simulink model "ResidualsGen"  (Simulink 9.3)
settings: Solver=ode23tb  StartTime=0.0  StopTime=1219  EnableMultiTasking=on
values from neighbouring files (symbols this model uses):
  omega_min = TC_ENGINE.turbo.omega_min    [RunEngine.m]
settings Model: Creator=nkymark  LastModifiedBy=markng
settings SolverCC: MaxConsecutiveMinStep=100  ZeroCrossControl=EnableAll  SolverResetMethod=Robust
settings DataIOCC: LimitDataPoints=on
settings DebuggingCC: AllowSymbolicDim=off  PregeneratedLibrarySubsystemCodeDiagnostic=none
settings SFSimCC: SimParseCustomCode=off
settings GRTTargetCC: GeneratePreprocessorConditionals=Disable all

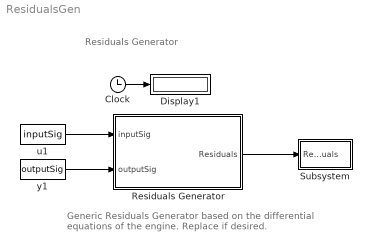
== system ResidualsGen ==
  note: Residuals Generator
  note: Generic Residuals Generator based on the differential
      | equations of the engine. Replace if desired.
  Clock : Clock
  Display1 : Display
  Residuals Generator : Subsystem
  Subsystem : Subsystem
  u1 : FromWorkspace  VariableName=inputSig  SampleTime=0
  y1 : FromWorkspace  VariableName=outputSig  SampleTime=0
  wires:
  Clock/1 -> Display1/1
  Residuals Generator/1(Residuals) -> Subsystem/1(Residuals)
  y1/1 -> Residuals Generator/2(outputSig)
  u1/1 -> Residuals Generator/1(inputSig)

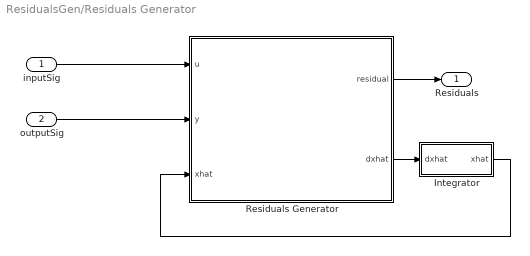
== system ResidualsGen/Residuals Generator ==
  inputSig : Inport
  outputSig : Inport  Port=2
  Integrator : Subsystem
  Residuals Generator : MATLAB Function  TreatAsAtomicUnit=on
  Residuals : Outport
  wires:
  inputSig/1 -> Residuals Generator/1(u)
  Integrator/1(xhat) -> Residuals Generator/3(xhat)
  Residuals Generator/1(residual) -> Residuals/1
  outputSig/1 -> Residuals Generator/2(y)
  Residuals Generator/2(dxhat) -> Integrator/1(dxhat)

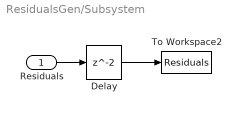
== system ResidualsGen/Subsystem ==
  Residuals : Inport
  Delay : Delay  SampleTime=0.1
  To Workspace2 : ToWorkspace  VariableName=Residuals  SaveFormat=Timeseries  SampleTime=-1
  wires:
  Residuals/1 -> Delay/1
  Delay/1 -> To Workspace2/1

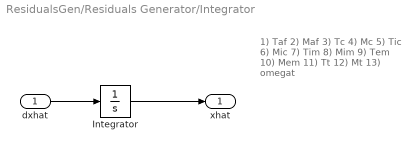
== system ResidualsGen/Residuals Generator/Integrator ==
  note: 1) Taf
      |  2) Maf
      |  3) Tc
      |  4) Mc
      |  5) Tic
      |  6) Mic
      |  7) Tim
      |  8) Mim
      |  9) Tem
      | 10) Mem
      | 11) Tt
      | 12) Mt
      | 13) omegat
  dxhat : Inport
  Integrator : Integrator  InitialCondition=[293 0.012002433760826 293 0.006001216 293 0.006001216 293 0.002160438 900 0.001005747 293 0.023773096 3000];  LimitOutput=on  UpperSaturationLimit=[inf inf inf inf inf inf inf inf inf inf inf inf 24000]  LowerSaturationLimit=-[inf inf inf inf inf inf inf inf inf inf inf inf -omega_min]  ZeroCross=off
  xhat : Outport
  wires:
  Integrator/1 -> xhat/1
  dxhat/1 -> Integrator/1

== matlab function Residuals Generator/Residuals Generator ==
  data: residual output double; u input double; y input double; xhat input double; dxhat output double
% This file descrtibes the model of the engine system via the dynamical equations. The equations can
% be found in the paper by Lars Eriksson (2007). 
%
%           [residual, dxhat] = Observer( u, y, xhat )
% 
% 
% The function takes in the control input 'u' and sensor output from the Simulink model in
% 'Engine.mdl'. By comparing the estimated output of the model based on the equations in this file
% with 'y', the 'Residual' is produced by computing r = \hat y - y.
% 
% 
% (C) Mark Ng, 2019
% Ulster University, UK
%
function [residual, dxhat] = Observer( u, y, xhat )

%#codegen
Vic = 0.005;
Vaf = 0.01;
Vim = 0.0018;
Vem = 0.0025;
Vex = 0.02;
AFs = 15.1;
Ra  = 287.2;
Rc  = 0.06;
Rem = 290;
rc  = 9.5;
Ce  = 0.8;
T0  = 1100;
Ceo = 3000;
cpc = 1.0052e+03;
Hic = 400000000;
Haf = 200000000;
Hex = 300000000;
lambda  = 1;
kappaic = 1.4;
kappath = 2;
kappaem = 1.3;
Diaem   = 0.04;
Diatc   = 0.05;
Lenem   = 0.45;
Pipeem  = 4;
muem    = 4.0000e-05;
MSem    = [0.26 0.6 0 0];
h_ext   = 95;
dampt   = 1.0000e-06;
inertt  = 3.0000e-05;
Psi_max = 2.3;
Phi_max = 0.12;
pic_lin = 500;
paf_lin = 2000;
pex_lin = 300;
epsilon = 0.8;
cvi     = Ra / (kappaic - 1);
cve     = Rem / (kappaem - 1);
cpeg    = 1.2567e+03;
cptc    = 1200;
cdwg    = 3.1500e-04;
k1tc    = 0.017;
k2tc    = 1.4;
etac_max    = 0.8;
Phic_etamax = 0.06;
lambdaem    = 0.07;
omegatmax   = 24000;

% if fault == 3
%     omegatmin = 200;
% else
%     omegatmin   = 2000;
% end

omegatmin = 2000;

tceff_max   = 0.75;
tceff_min   = 0.3;
BSReff_max  = 0.7;


%%%%%%%%%%%%%%%%%%%%%%%%%%%%%%%%%%%%%%%%%%%%%%%%%%%%%%%%%
% Establishment of inputs
xth    = u(1);   % xth
omegae = u(2);   % omegae (rad/s)
xwg    = u(3);   % xwg
pamb   = u(4);   % pamb
Tamb   = u(5);   % Tamb

%%%%%%%%%%%%%%%%%%%%%%%%%%%%%%%%%%%%%%%%%%%%%%%%%%%%%%%%%
% Establishment of states
Taf = xhat(1);
Maf = xhat(2);
Tc  = xhat(3);
Mc  = xhat(4);
Tic = xhat(5);
Mic = xhat(6);
Tim = xhat(7);
Mim = xhat(8);
Tem = xhat(9);
Mem = xhat(10);
Tt  = xhat(11);
Mt  = xhat(12);
omegat = xhat(13);

paf = Taf * Ra * Maf / Vaf;
pc = Tc * Ra * Mc / Vic;
pic = Tic * Ra * Mic / Vic;
pim  = (Tim * Ra *  Mim / Vim);
pem  = Tem * Rem * Mem / Vem;
pt   = Tt  * Rem * Mt  / Vex;

if omegat < omegatmin
    omegat = omegatmin;
elseif omegat > omegatmax
    omegat = omegatmax;
end

%%%%%%%%%%%%%%%%%%%%%%%%%%%%%%%%%%%%%%%%%%%%%%%%%%%%%%%%%
Tus_af  = 0;
pus_af  = 0;
pds_af  = 0;
Hin_af1 = 0;
Hin_af2 = 0;

if (pamb < paf) + 1 == 1
    pus_af = pamb;
    pds_af = paf;
    Tus_af = Tamb;
elseif (pamb < paf) + 1 == 2
    pds_af = pamb;
    pus_af = paf;
    Tus_af = Taf;
end
Tflow_af = Tus_af;

signp_af = sign( pamb - paf );
Hin_af2  = sqrt( abs( pus_af / (Haf * Tus_af) ) );
if (paf_lin > (pus_af - pds_af)) + 1 == 1
    Hin_af1 = sqrt( abs( pus_af - pds_af ) );
elseif (paf_lin > (pus_af - pds_af)) + 1 == 2
    Hin_af1 = (pus_af - pds_af) / sqrt( paf_lin );
end
Waf = Hin_af1 * Hin_af2 * signp_af;

% Solving for PIc
PIc = (pc / paf);
if PIc < 1
    PIc = 1;
elseif PIc > 10
    PIc = 10;
end

% Solving for Wc
Psic    = (PIc^((kappaic - 1) / kappaic) - 1) * (cpc / Rc^2) * Taf / ((omegat / (2 * pi))^2);
Psicnew = (Psic / Psi_max)^2;
if Psicnew < 0
    Psicnew = 0;
elseif Psicnew > 1
    Psicnew = 1;
end
Phic    = sqrt( abs( 1 - Psicnew ) ) * Phi_max;
Wc      = Phic * Rc^3 * (omegat / (2 * pi)) * paf / (Taf * Ra);

% Solving for dTaf
dTaf = ((Tflow_af * Waf * (Ra + cvi)) - (Taf * Wc * (Ra + cvi)) - (cvi * (Waf - Wc) * Taf)) / (cvi * Maf);

% Solving for paf
dMaf = Waf - Wc;


%%%%%%%%%%%%%%%%%%%%%%%%%%%%%%%%%%%%%%%%%%%%%%%%%%%%%%%%%
% Solving for etac
Phiceta = Wc / Rc^3 / (omegat / (2 * pi)) / (paf / (Taf * Ra));
etac   = Phiceta * (2 * Phic_etamax - Phiceta) * (etac_max / Phic_etamax^2);
if etac < 0.3
    etac = 0.3;
elseif etac > 1
    etac = 1;
end

% Solving for Tc1
PIc2 = pc / paf;
if PIc2 < 1
    PIc2 = 1;
end
Tc1  = (((PIc2^(1 - 1 / kappaic) - 1) / etac) + 1) * Taf;

% Solving for Tqc
Tc2 = Tc1 - Taf;
if Tc2 < 0
    Tc2 = 0;
end
Tqc = Tc2 * Wc * 1100 / omegat;

Tus_ic  = 0;
pus_ic  = 0;
pds_ic  = 0;
Hin_ic1 = 0;
Hin_ic2 = 0;

% Solving for Wic
if (pc < pic) + 1 == 1
    pus_ic = pc;
    pds_ic = pic;
    Tus_ic = Tc;
elseif (pc < pic) + 1 == 2
    pds_ic = pc;
    pus_ic = pic;
    Tus_ic = Tic;
end
Tflow_ic = Tus_ic;
signp_ic = sign( pc - pic );
Hin_ic2  = sqrt( abs( pus_ic / (Hic * Tus_ic) ) );
if (pic_lin > (pus_ic - pds_ic)) + 1 == 1
    Hin_ic1 = sqrt( abs( pus_ic - pds_ic ) );
elseif (pic_lin > (pus_ic - pds_ic)) + 1 == 2
    Hin_ic1 = (pus_ic - pds_ic) / sqrt( pic_lin );
end
Wic = Hin_ic1 * Hin_ic2 * signp_ic;

% Solving for dTc
dTc = ((Tc1 * Wc * (Ra + cvi)) - (Tc * Wic * (Ra + cvi)) - (cvi * (Wc - Wic) * Tc)) / (cvi * Mc);

% Solving for dpc
dMc = Wc - Wic;


%%%%%%%%%%%%%%%%%%%%%%%%%%%%%%%%%%%%%%%%%%%%%%%%%%%%%%%%%
% Solving for Tflow
Tflow = Tflow_ic - (epsilon * (Tflow_ic - Tamb));

Tus_th  = 0;
pus_th  = 0;
pds_th  = 0;
Hin_th1 = 0;
Hin_th2 = 0;

% Solving for Wth
if (pic < pim) + 1 == 1
    pus_th = pic;
    pds_th = pim;
    Tus_th = Tic;
elseif (pic < pim) + 1 == 2
    pds_th = pic;
    pus_th = pim;
    Tus_th = Tim;
end
Tflow_th = Tus_th;

signp_th = sign( pic - pim );
Hin_th2  = pus_th * xth / sqrt( abs( Tus_th * Ra ) );
if (pds_th / pus_th) > ((2 / (kappath + 1))^(kappath / (kappath - 1)))
    Hin_th1a = (pds_th / pus_th);
else
    Hin_th1a = ((2 / (kappath + 1))^(kappath / (kappath - 1)));
end
Hin_th1b = Hin_th1a^(2 / kappath) - Hin_th1a^((kappath + 1) / kappath);
Hin_th1  = sqrt( abs( Hin_th1b * (2 * kappath / (kappath - 1)) ) );
Wth = Hin_th1 * Hin_th2 * signp_th;

% Solving for Tth
Tth  = Tflow_th;

% Solving for dTic
dTic = ((Wic * Tflow * (Ra + cvi)) - (Tth * Wth * (Ra + cvi)) - (cvi * (Wic - Wth) * Tic)) / (cvi * Mic);

% Solving for dpic
dMic = Wic - Wth;


%%%%%%%%%%%%%%%%%%%%%%%%%%%%%%%%%%%%%%%%%%%%%%%%%%%%%%%%%
% Solving for Wei
Wei = pim * (rc - (abs( pem / pim ))^(1 / kappaem)) * (Ce / (rc - 1)) * (Vim / 4 / pi / Ra) * omegae / Tim;

% Solving for Wf
Wf  = Wei / (AFs * lambda);

% Solving for Weo
Weo = Wei + Wf;

% Solving for Teo
Teo = (Weo * Ceo) + T0;

h_int = 0.7^MSem(3) * ((4 / (pi * Diaem * muem)) * (abs( Weo / Pipeem )))^MSem(2) * MSem(1) / (Diaem / lambdaem);
h_tot = 1 / ((1 / h_ext) + (1 / h_int));
Tti   = Tamb + ((Teo - Tamb) * exp(- (h_tot * pi * Diaem * Lenem) / (Weo / Pipeem) / (Rem * kappaem / (kappaem - 1))));

% Solving for dTim
dTim = ((Tth * Wth * (Ra + cvi)) - (Tim * Wei * (Ra + cvi)) - (cvi * (Wth - Wei) * Tim)) / (cvi * Mim);

% Solving for dpim
dMim = Wth - Wei;


%%%%%%%%%%%%%%%%%%%%%%%%%%%%%%%%%%%%%%%%%%%%%%%%%%%%%%%%%
% Solving for Torque of Engine
Gross    = (Wf * 44e6 * 0.41 * min( 1,(Wei / (AFs * Wf)) ) / (0.25 / pi * omegae)) * 0.25 / pi;
Friction1= omegae * (4 * Vim / Pipeem / 0.09^2 / pi^2);
Friction2= ( (0.464 + 0.0072 * Friction1^1.8) * 1.5 ) + ( ( (Wei / ( Vim * omegae * (1 / (4 * pi) ) ) * 1.2e6) - 0.2e6 ) * 0.0215 );
Friction = Friction2 * sqrt( 75/(0.09 * 1e3) ) * 1.3 * Vim * 0.25 / pi;
Pumping  = (pem - pim) * Vim * 0.25 / pi;
Tq_eEST   = Gross - Friction - Pumping; 
if Tq_eEST > 350 
    Tq_eEST = 350;
elseif Tq_eEST < 1
    Tq_eEST = 1;
end


%%%%%%%%%%%%%%%%%%%%%%%%%%%%%%%%%%%%%%%%%%%%%%%%%%%%%%%%%
Tus_wg  = 0;
pus_wg  = 0;
pds_wg  = 0;
Hin_wg1 = 0;
Hin_wg2 = 0;

% Solving for Wwg
if (pem < pt) + 1 == 1
    pus_wg = pem;
    pds_wg = pt;
    Tus_wg = Tem;
elseif (pem < pt) + 1 == 2
    pds_wg = pem;
    pus_wg = pt;
    Tus_wg = Tt;
end
Tflow_wg = Tus_wg;
signp_wg = sign( pem - pt );
Hin_wg2  = pus_wg * xwg * cdwg / sqrt( abs( Tus_wg * Rem ) );
if (pds_wg / pus_wg) > ((2 / (kappaem + 1))^(kappaem / (kappaem - 1)))
    Hin_wg1a = (pds_wg / pus_wg);
else
    Hin_wg1a = ((2 / (kappaem + 1))^(kappaem / (kappaem - 1)));
end
Hin_wg1b = Hin_wg1a^(2 / kappaem) - Hin_wg1a^((kappaem + 1) / kappaem);
Hin_wg1  = sqrt( abs( Hin_wg1b) * (2 * kappaem / (kappaem - 1) ) );
Wwg      = Hin_wg1 * Hin_wg2 * signp_wg;

% Solving for PIt
PIt = min( pt / pem,1 );

% Solving for etat
BSR1 = (1 - abs( 1 / PIt )^((1 - kappaem) / kappaem)) * 2 * cpeg * Tem;
BSR  = omegat / sqrt( max( BSR1,0.001 ) ) * (Diatc / 2);
etat = tceff_max * (1 - ((BSR - BSReff_max) / BSReff_max)^2);
if etat <= tceff_min
    etat = tceff_min;
elseif etat >= tceff_max
        etat = tceff_max;
end

% Solving for Tto
Tto  = Tem * (1 - etat * (1 - abs( PIt )^(1 - 1 / kappaem)));

% Solving for Wt
Wt1 = max( 1 - abs( PIt )^k2tc,0 );
Wt  = sqrt( abs( Wt1 ) ) * k1tc * pem * 1e-3 / sqrt( abs( Tem ) );

% Solving for Tqt
Tqt1 = max( Tem - Tto,0 );
Tqt  = Tqt1 * Wt * cptc / omegat;

% Solving for Wes
Wes  = -(Wt + Wwg);

% Solving for dTem
dTem = ((Tem * Wes * (Rem + cve)) - (Tti * (-Weo) * (Rem + cve)) - (cve * (Wes - (-Weo)) * Tem)) / (cve * Mem);

% Solving for dpem
dMem = Wes - (-Weo);

% Solving for domegat 
domegat = ((Tqt - Tqc) - (dampt * omegat)) / inertt;


% %%%%%%%%%%%%%%%%%%%%%%%%%%%%%%%%%%%%%%%%%%%%%%%%%%%%%%%%%
% % Solving for Tturbo
Tturbo  = ((Wt * cpeg * Tto) + (Wwg * cpeg * Tflow_wg)) / ((Wt * cpeg) + (Wwg * cpeg)); 

Tus_exh  = 0;
pus_exh  = 0;
pds_exh  = 0;
Hin_exh1 = 0;
Hin_exh2 = 0;

% Solving for Wesfinal
if (pamb < pt) + 1 == 1
    pus_exh = pamb;
    pds_exh = pt;
    Tus_exh = Tamb;
elseif (pamb < pt) + 1 == 2
    pds_exh = pamb;
    pus_exh = pt;
    Tus_exh = Tt;
end
Tflow_exh = Tus_exh;
signp_exh = sign( pamb - pt );
Hin_exh2  = sqrt( abs( pus_exh / (Hex * Tus_exh) ) );
if (pex_lin > (pus_exh - pds_exh)) + 1 == 1
    Hin_exh1 = sqrt( pus_exh - pds_exh );
elseif (pex_lin > (pus_exh - pds_exh)) + 1 == 2
    Hin_exh1 = (pus_exh - pds_exh) / sqrt( pex_lin );
end
Wesfinal = Hin_exh1 * Hin_exh2 * signp_exh;

% Solving for dTt
dTt = ((Tflow_exh * Wesfinal * (Rem + cve)) - (Tturbo * Wes * (Rem + cve)) - (cve * (Wesfinal - Wes) * Tt)) / (cve * Mt);

% Solving for dpt
dMt  = Wesfinal - Wes;

residual = ( [Tc; pc; Tic; pic; Tim; pim; Waf; Tq_eEST; pem] - [y(1); y(2); y(3); y(4); y(5); y(6); y(7); y(8); y(9)]);

dxhat    = [dTaf dMaf dTc dMc dTic dMic dTim dMim dTem dMem dTt dMt domegat];
